simulink model "gradingSystem"  (R2018b)
settings: Solver=FixedStepDiscrete  StartTime=0.0  StopTime=10.0  RelTol=1e-3
settings Model: Creator=asmaa  LastModifiedBy=asmaa
settings OptimizationCC: DefaultParameterBehavior=Inlined  EnhancedBackFolding=on  PassReuseOutputArgsAs=Individual arguments  OptimizeBlockOrder=speed  DifferentSizesBufferReuse=on  OptimizationCustomize=off
settings DebuggingCC: UnderspecifiedInitializationDetection=Classic  MergeDetectMultiDrivingBlocksExec=none  ParameterTunabilityLossMsg=error
settings ModelReferenceCC: PropagateSignalLabelsOutOfModel=off
settings SFSimCC: MATLABDynamicMemAlloc=off
settings RTWCC: SystemTargetFile=ert.tlc  GenCodeOnly=on  TemplateMakefile=ert_default_tmf  GenerateReport=on  IncludeHyperlinkInReport=on  LaunchReport=on  GenerateTraceInfo=on  GenerateTraceReport=on  GenerateTraceReportSl=on  GenerateTraceReportSf=on  GenerateTraceReportEml=on
settings CodeAppCC: ForceParamTrailComments=on  IgnoreCustomStorageClasses=off  OperatorAnnotations=on  SimulinkDataObjDesc=on  SFDataObjDesc=on  InsertBlockDesc=on
settings ERTTargetCC: TargetLangStandard=C99 (ISO)  GenerateSampleERTMain=on  InlinedParameterPlacement=NonHierarchical  ERTCustomFileTemplate=example_file_process.tlc

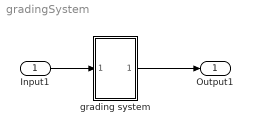
== system gradingSystem ==
  "Input1 " : Inport
  grading system : Subsystem
  "Output1 " : Outport
  wires:
  "Input1 "/1 -> grading system/1(In1)
  grading system/1(Out1) -> "Output1 "/1

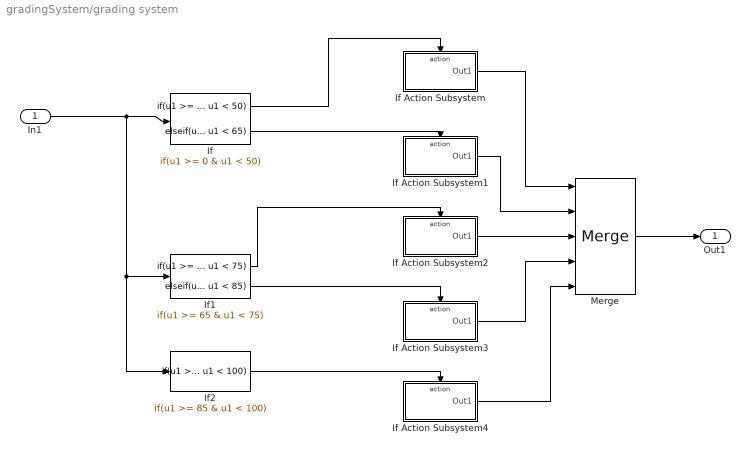
== system gradingSystem/grading system ==
  In1 : Inport
  If : If  IfExpression=u1 >= 0 & u1 < 50  ElseIfExpressions=u1 >= 50 & u1 < 65  ShowElse=off
  If Action Subsystem : Subsystem  TreatAsAtomicUnit=on
  If Action Subsystem1 : Subsystem  TreatAsAtomicUnit=on
  If Action Subsystem2 : Subsystem  TreatAsAtomicUnit=on
  If Action Subsystem3 : Subsystem  TreatAsAtomicUnit=on
  If Action Subsystem4 : Subsystem  TreatAsAtomicUnit=on
  If1 : If  IfExpression=u1 >= 65 & u1 < 75  ElseIfExpressions=u1 >= 75 & u1 < 85  ShowElse=off
  If2 : If  IfExpression=u1 >= 85 & u1 < 100  ShowElse=off
  Merge : Merge  Inputs=5
  Out1 : Outport
  wires:
  In1/1 -> If2/1, If1/1, If/1
  If2/1 -> If Action Subsystem4/Action
  Merge/1 -> Out1/1
  If Action Subsystem2/1(Out1) -> Merge/3
  If Action Subsystem3/1(Out1) -> Merge/4
  If Action Subsystem1/1(Out1) -> Merge/2
  If Action Subsystem/1(Out1) -> Merge/1
  If Action Subsystem4/1(Out1) -> Merge/5
  If/2 -> If Action Subsystem1/Action
  If1/2 -> If Action Subsystem3/Action
  If/1 -> If Action Subsystem/Action
  If1/1 -> If Action Subsystem2/Action

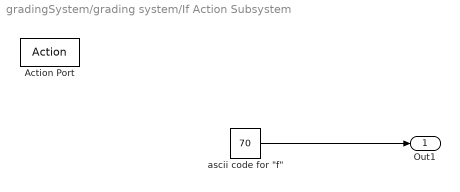
== system gradingSystem/grading system/If Action Subsystem ==
  Action Port : ActionPort  ActionType=then
  "ascii code for \"f\"" : Constant  Value=70  OutDataTypeStr=uint8
  Out1 : Outport
  wires:
  "ascii code for \"f\""/1 -> Out1/1

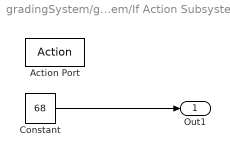
== system gradingSystem/grading system/If Action Subsystem1 ==
  Action Port : ActionPort  ActionType=elseif
  Constant : Constant  Value=68  OutDataTypeStr=uint8
  Out1 : Outport
  wires:
  Constant/1 -> Out1/1

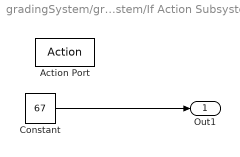
== system gradingSystem/grading system/If Action Subsystem2 ==
  Action Port : ActionPort  ActionType=then
  Constant : Constant  Value=67  OutDataTypeStr=uint8
  Out1 : Outport
  wires:
  Constant/1 -> Out1/1

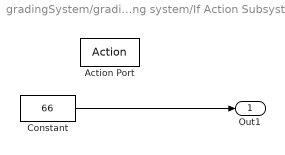
== system gradingSystem/grading system/If Action Subsystem3 ==
  Action Port : ActionPort  ActionType=elseif
  Constant : Constant  Value=66  OutDataTypeStr=uint8
  Out1 : Outport
  wires:
  Constant/1 -> Out1/1

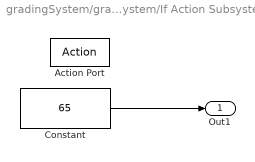
== system gradingSystem/grading system/If Action Subsystem4 ==
  Action Port : ActionPort  ActionType=then
  Constant : Constant  Value=65  OutDataTypeStr=uint8  LockScale=on
  Out1 : Outport
  wires:
  Constant/1 -> Out1/1
